simulink library "Quat2Euler"  (Simulink 7.2)
settings: Solver=ode45  StartTime=0.0  StopTime=10.0  RelTol=1e-3
settings Model: Creator=matlab  LastModifiedBy=matlab

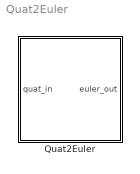
== system Quat2Euler ==
  Quat2Euler : Subsystem  mask(Quat2Euler){euler_order=321, quat_convention=1}
      mask prompts: euler_order "Euler angle order"; quat_convention "Quaternion scalar convention"
      mask help: Convert quaternion to Euler angles
      mask StyleString: popup(312|321|123|132|231|213|121|131|212|232|313|323),popup(1|4)

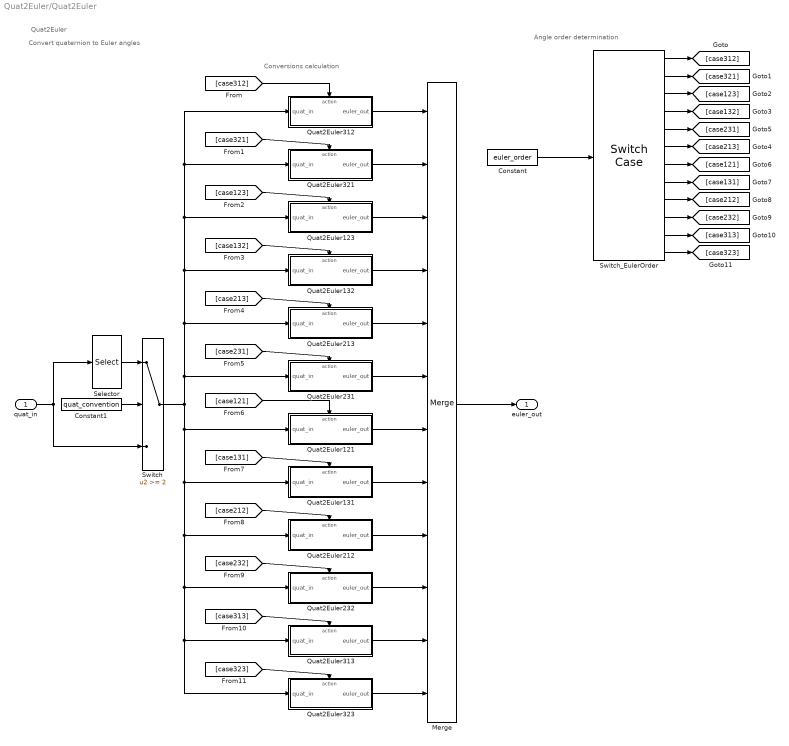
== system Quat2Euler/Quat2Euler ==
  note: Quat2Euler
  note: Convert quaternion to Euler angles
  note: Angle order determination
  note: Conversions calculation
  quat_in : Inport  Description=[ ]: Input quaternion.  PortDimensions=4  OutDataType=sfix(16)  OutScaling=2^0
  Constant : Constant  Value=euler_order  OutDataType=sfix(16)  OutScaling=2^0
  Constant1 : Constant  Value=quat_convention  OutDataType=sfix(16)  OutScaling=2^0
  Merge : Merge  Inputs=12
  Quat2Euler121 : Subsystem  TreatAsAtomicUnit=on
  Quat2Euler123 : Subsystem  TreatAsAtomicUnit=on
  Quat2Euler131 : Subsystem  TreatAsAtomicUnit=on
  Quat2Euler132 : Subsystem  TreatAsAtomicUnit=on
  Quat2Euler212 : Subsystem  TreatAsAtomicUnit=on
  Quat2Euler213 : Subsystem  TreatAsAtomicUnit=on
  Quat2Euler231 : Subsystem  TreatAsAtomicUnit=on
  Quat2Euler232 : Subsystem  TreatAsAtomicUnit=on
  Quat2Euler312 : Subsystem  TreatAsAtomicUnit=on
  Quat2Euler313 : Subsystem  TreatAsAtomicUnit=on
  Quat2Euler321 : Subsystem  TreatAsAtomicUnit=on
  Quat2Euler323 : Subsystem  TreatAsAtomicUnit=on
  Selector : Selector  InputPortWidth=4  IndexOptions=Index vector (dialog)  Indices=[4 1 2 3]  OutputSizes=1
  Switch : Switch  Threshold=2  OutDataType=sfix(16)  OutScaling=2^0
  Switch_EulerOrder : SwitchCase  CaseConditions={1,2,3,4,5,6,7,8,9,10,11,12}  CaseShowDefault=off
  euler_out : Outport  Description=[rad]: Eqivalent Euler angles.  PortDimensions=3  OutDataType=sfix(16)  OutScaling=2^0
  wires:
  Merge/1 -> euler_out/1
  Switch/1 -> Quat2Euler121/1(quat_in), Quat2Euler131/1(quat_in), Quat2Euler212/1(quat_in), Quat2Euler232/1(quat_in), Quat2Euler323/1(quat_in), Quat2Euler313/1(quat_in), Quat2Euler231/1(quat_in), Quat2Euler213/1(quat_in), Quat2Euler132/1(quat_in), Quat2Euler123/1(quat_in), Quat2Euler321/1(quat_in), Quat2Euler312/1(quat_in)
  quat_in/1 -> Switch/3, Selector/1
  Constant1/1 -> Switch/2
  Selector/1 -> Switch/1
  Quat2Euler121/1(euler_out) -> Merge/7
  Quat2Euler312/1(euler_out) -> Merge/1
  Quat2Euler321/1(euler_out) -> Merge/2
  Quat2Euler123/1(euler_out) -> Merge/3
  Quat2Euler132/1(euler_out) -> Merge/4
  Quat2Euler213/1(euler_out) -> Merge/5
  Quat2Euler231/1(euler_out) -> Merge/6
  Quat2Euler131/1(euler_out) -> Merge/8
  Quat2Euler212/1(euler_out) -> Merge/9
  Quat2Euler232/1(euler_out) -> Merge/10
  Quat2Euler313/1(euler_out) -> Merge/11
  Quat2Euler323/1(euler_out) -> Merge/12
  [case121] -> Quat2Euler121/Action
  [case131] -> Quat2Euler131/Action
  [case212] -> Quat2Euler212/Action
  [case232] -> Quat2Euler232/Action
  [case313] -> Quat2Euler313/Action
  [case323] -> Quat2Euler323/Action
  Switch_EulerOrder/12 -> [case323]
  Switch_EulerOrder/11 -> [case313]
  Switch_EulerOrder/10 -> [case232]
  Switch_EulerOrder/9 -> [case212]
  Switch_EulerOrder/8 -> [case131]
  Switch_EulerOrder/7 -> [case121]
  Switch_EulerOrder/5 -> [case231]
  Switch_EulerOrder/6 -> [case213]
  Constant/1 -> Switch_EulerOrder/1
  Switch_EulerOrder/1 -> [case312]
  Switch_EulerOrder/3 -> [case123]
  Switch_EulerOrder/2 -> [case321]
  Switch_EulerOrder/4 -> [case132]
  [case312] -> Quat2Euler312/Action
  [case321] -> Quat2Euler321/Action
  [case123] -> Quat2Euler123/Action
  [case132] -> Quat2Euler132/Action
  [case213] -> Quat2Euler213/Action
  [case231] -> Quat2Euler231/Action

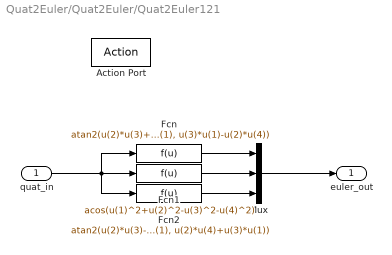
== system Quat2Euler/Quat2Euler/Quat2Euler121 ==
  quat_in : Inport  OutDataType=sfix(16)  OutScaling=2^0
  Action Port : ActionPort
  Fcn : Fcn  Expr=atan2(u(2)*u(3)+u(4)*u(1), u(3)*u(1)-u(2)*u(4))
  Fcn1 : Fcn  Expr=acos(u(1)^2+u(2)^2-u(3)^2-u(4)^2)
  Fcn2 : Fcn  Expr=atan2(u(2)*u(3)-u(4)*u(1), u(2)*u(4)+u(3)*u(1))
  Mux : Mux  Inputs=3
  euler_out : Outport  OutDataType=sfix(16)  OutScaling=2^0
  wires:
  Mux/1 -> euler_out/1
  quat_in/1 -> Fcn2/1, Fcn/1, Fcn1/1
  Fcn2/1 -> Mux/3
  Fcn1/1 -> Mux/2
  Fcn/1 -> Mux/1

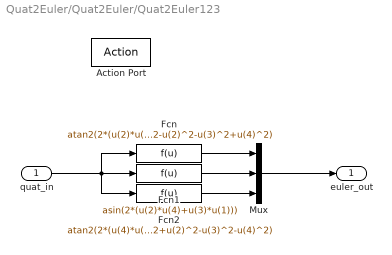
== system Quat2Euler/Quat2Euler/Quat2Euler123 ==
  quat_in : Inport  OutDataType=sfix(16)  OutScaling=2^0
  Action Port : ActionPort
  Fcn : Fcn  Expr=atan2(2*(u(2)*u(1)-u(3)*u(4)),u(1)^2-u(2)^2-u(3)^2+u(4)^2)
  Fcn1 : Fcn  Expr=asin(2*(u(2)*u(4)+u(3)*u(1)))
  Fcn2 : Fcn  Expr=atan2(2*(u(4)*u(1)-u(2)*u(3)),u(1)^2+u(2)^2-u(3)^2-u(4)^2)
  Mux : Mux  Inputs=3
  euler_out : Outport  OutDataType=sfix(16)  OutScaling=2^0
  wires:
  Mux/1 -> euler_out/1
  quat_in/1 -> Fcn2/1, Fcn/1, Fcn1/1
  Fcn2/1 -> Mux/3
  Fcn1/1 -> Mux/2
  Fcn/1 -> Mux/1

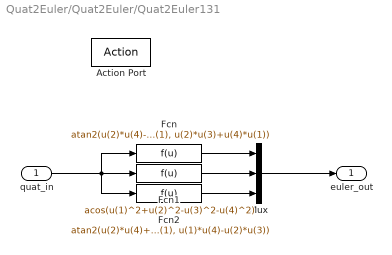
== system Quat2Euler/Quat2Euler/Quat2Euler131 ==
  quat_in : Inport  OutDataType=sfix(16)  OutScaling=2^0
  Action Port : ActionPort
  Fcn : Fcn  Expr=atan2(u(2)*u(4)-u(3)*u(1), u(2)*u(3)+u(4)*u(1))
  Fcn1 : Fcn  Expr=acos(u(1)^2+u(2)^2-u(3)^2-u(4)^2)
  Fcn2 : Fcn  Expr=atan2(u(2)*u(4)+u(3)*u(1), u(1)*u(4)-u(2)*u(3))
  Mux : Mux  Inputs=3
  euler_out : Outport  OutDataType=sfix(16)  OutScaling=2^0
  wires:
  Fcn/1 -> Mux/1
  Fcn1/1 -> Mux/2
  Fcn2/1 -> Mux/3
  quat_in/1 -> Fcn1/1, Fcn/1, Fcn2/1
  Mux/1 -> euler_out/1

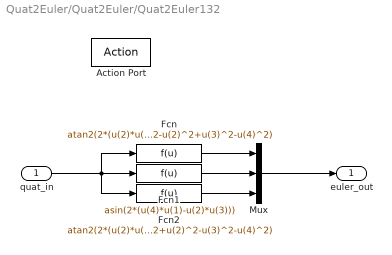
== system Quat2Euler/Quat2Euler/Quat2Euler132 ==
  quat_in : Inport  OutDataType=sfix(16)  OutScaling=2^0
  Action Port : ActionPort
  Fcn : Fcn  Expr=atan2(2*(u(2)*u(1)+u(3)*u(4)),u(1)^2-u(2)^2+u(3)^2-u(4)^2)
  Fcn1 : Fcn  Expr=asin(2*(u(4)*u(1)-u(2)*u(3)))
  Fcn2 : Fcn  Expr=atan2(2*(u(2)*u(4)+u(3)*u(1)),u(1)^2+u(2)^2-u(3)^2-u(4)^2)
  Mux : Mux  Inputs=3
  euler_out : Outport  OutDataType=sfix(16)  OutScaling=2^0
  wires:
  Fcn/1 -> Mux/1
  Fcn1/1 -> Mux/2
  Fcn2/1 -> Mux/3
  quat_in/1 -> Fcn1/1, Fcn/1, Fcn2/1
  Mux/1 -> euler_out/1

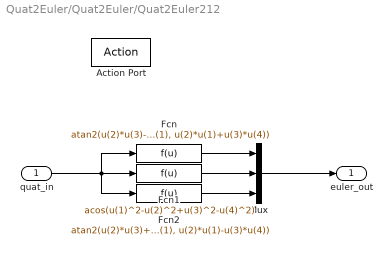
== system Quat2Euler/Quat2Euler/Quat2Euler212 ==
  quat_in : Inport  OutDataType=sfix(16)  OutScaling=2^0
  Action Port : ActionPort
  Fcn : Fcn  Expr=atan2(u(2)*u(3)-u(4)*u(1), u(2)*u(1)+u(3)*u(4))
  Fcn1 : Fcn  Expr=acos(u(1)^2-u(2)^2+u(3)^2-u(4)^2)
  Fcn2 : Fcn  Expr=atan2(u(2)*u(3)+u(4)*u(1), u(2)*u(1)-u(3)*u(4))
  Mux : Mux  Inputs=3
  euler_out : Outport  OutDataType=sfix(16)  OutScaling=2^0
  wires:
  Mux/1 -> euler_out/1
  quat_in/1 -> Fcn2/1, Fcn/1, Fcn1/1
  Fcn2/1 -> Mux/3
  Fcn1/1 -> Mux/2
  Fcn/1 -> Mux/1

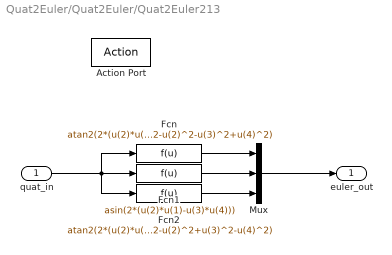
== system Quat2Euler/Quat2Euler/Quat2Euler213 ==
  quat_in : Inport  OutDataType=sfix(16)  OutScaling=2^0
  Action Port : ActionPort
  Fcn : Fcn  Expr=atan2(2*(u(2)*u(4)+u(3)*u(1)),u(1)^2-u(2)^2-u(3)^2+u(4)^2)
  Fcn1 : Fcn  Expr=asin(2*(u(2)*u(1)-u(3)*u(4)))
  Fcn2 : Fcn  Expr=atan2(2*(u(2)*u(3)+u(4)*u(1)),u(1)^2-u(2)^2+u(3)^2-u(4)^2)
  Mux : Mux  Inputs=3
  euler_out : Outport  OutDataType=sfix(16)  OutScaling=2^0
  wires:
  Mux/1 -> euler_out/1
  quat_in/1 -> Fcn2/1, Fcn/1, Fcn1/1
  Fcn2/1 -> Mux/3
  Fcn1/1 -> Mux/2
  Fcn/1 -> Mux/1

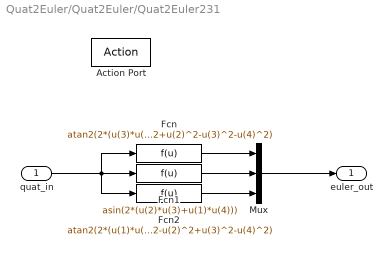
== system Quat2Euler/Quat2Euler/Quat2Euler231 ==
  quat_in : Inport  OutDataType=sfix(16)  OutScaling=2^0
  Action Port : ActionPort
  Fcn : Fcn  Expr=atan2(2*(u(3)*u(1)-u(4)*u(2)),u(1)^2+u(2)^2-u(3)^2-u(4)^2)
  Fcn1 : Fcn  Expr=asin(2*(u(2)*u(3)+u(1)*u(4)))
  Fcn2 : Fcn  Expr=atan2(2*(u(1)*u(2)-u(3)*u(4)),u(1)^2-u(2)^2+u(3)^2-u(4)^2)
  Mux : Mux  Inputs=3
  euler_out : Outport  OutDataType=sfix(16)  OutScaling=2^0
  wires:
  Fcn/1 -> Mux/1
  Fcn1/1 -> Mux/2
  Fcn2/1 -> Mux/3
  quat_in/1 -> Fcn1/1, Fcn/1, Fcn2/1
  Mux/1 -> euler_out/1

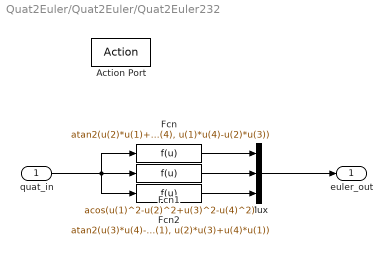
== system Quat2Euler/Quat2Euler/Quat2Euler232 ==
  quat_in : Inport  OutDataType=sfix(16)  OutScaling=2^0
  Action Port : ActionPort
  Fcn : Fcn  Expr=atan2(u(2)*u(1)+u(3)*u(4), u(1)*u(4)-u(2)*u(3))
  Fcn1 : Fcn  Expr=acos(u(1)^2-u(2)^2+u(3)^2-u(4)^2)
  Fcn2 : Fcn  Expr=atan2(u(3)*u(4)-u(2)*u(1), u(2)*u(3)+u(4)*u(1))
  Mux : Mux  Inputs=3
  euler_out : Outport  OutDataType=sfix(16)  OutScaling=2^0
  wires:
  Fcn/1 -> Mux/1
  Fcn1/1 -> Mux/2
  Fcn2/1 -> Mux/3
  quat_in/1 -> Fcn1/1, Fcn/1, Fcn2/1
  Mux/1 -> euler_out/1

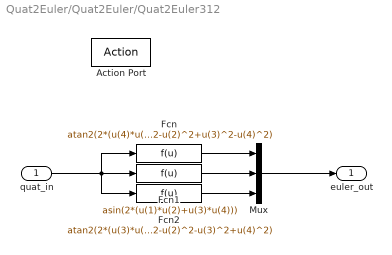
== system Quat2Euler/Quat2Euler/Quat2Euler312 ==
  quat_in : Inport  OutDataType=sfix(16)  OutScaling=2^0
  Action Port : ActionPort
  Fcn : Fcn  Expr=atan2(2*(u(4)*u(1)-u(2)*u(3)),u(1)^2-u(2)^2+u(3)^2-u(4)^2)
  Fcn1 : Fcn  Expr=asin(2*(u(1)*u(2)+u(3)*u(4)))
  Fcn2 : Fcn  Expr=atan2(2*(u(3)*u(1)-u(2)*u(4)),u(1)^2-u(2)^2-u(3)^2+u(4)^2)
  Mux : Mux  Inputs=3
  euler_out : Outport  OutDataType=sfix(16)  OutScaling=2^0
  wires:
  Mux/1 -> euler_out/1
  quat_in/1 -> Fcn2/1, Fcn/1, Fcn1/1
  Fcn2/1 -> Mux/3
  Fcn1/1 -> Mux/2
  Fcn/1 -> Mux/1

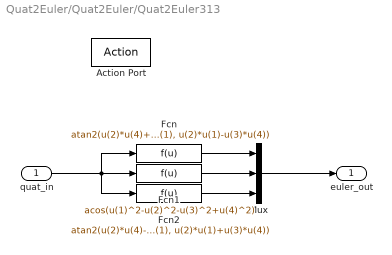
== system Quat2Euler/Quat2Euler/Quat2Euler313 ==
  quat_in : Inport  OutDataType=sfix(16)  OutScaling=2^0
  Action Port : ActionPort
  Fcn : Fcn  Expr=atan2(u(2)*u(4)+u(3)*u(1), u(2)*u(1)-u(3)*u(4))
  Fcn1 : Fcn  Expr=acos(u(1)^2-u(2)^2-u(3)^2+u(4)^2)
  Fcn2 : Fcn  Expr=atan2(u(2)*u(4)-u(3)*u(1), u(2)*u(1)+u(3)*u(4))
  Mux : Mux  Inputs=3
  euler_out : Outport  OutDataType=sfix(16)  OutScaling=2^0
  wires:
  Mux/1 -> euler_out/1
  quat_in/1 -> Fcn2/1, Fcn/1, Fcn1/1
  Fcn2/1 -> Mux/3
  Fcn1/1 -> Mux/2
  Fcn/1 -> Mux/1

== system Quat2Euler/Quat2Euler/Quat2Euler321 ==
  quat_in : Inport  OutDataType=sfix(16)  OutScaling=2^0
  Action Port : ActionPort
  Fcn : Fcn  Expr=atan2(2*(u(2)*u(3)+u(4)*u(1)),u(1)^2+u(2)^2-u(3)^2-u(4)^2)
  Fcn1 : Fcn  Expr=asin(2*(u(3)*u(1)-u(2)*u(4)))
  Fcn2 : Fcn  Expr=atan2(2*(u(2)*u(1)+u(4)*u(3)),u(1)^2-u(2)^2-u(3)^2+u(4)^2)
  Mux : Mux  Inputs=3
  euler_out : Outport  OutDataType=sfix(16)  OutScaling=2^0
  wires:
  Fcn/1 -> Mux/1
  Fcn1/1 -> Mux/2
  Fcn2/1 -> Mux/3
  quat_in/1 -> Fcn1/1, Fcn/1, Fcn2/1
  Mux/1 -> euler_out/1

== system Quat2Euler/Quat2Euler/Quat2Euler323 ==
  quat_in : Inport  OutDataType=sfix(16)  OutScaling=2^0
  Action Port : ActionPort
  Fcn : Fcn  Expr=atan2(u(3)*u(4)-u(1)*u(2), u(2)*u(4)+u(3)*u(1))
  Fcn1 : Fcn  Expr=acos(u(1)^2-u(2)^2-u(3)^2+u(4)^2)
  Fcn2 : Fcn  Expr=atan2(u(2)*u(1)+u(3)*u(4), u(3)*u(1)-u(2)*u(4))
  Mux : Mux  Inputs=3
  euler_out : Outport  OutDataType=sfix(16)  OutScaling=2^0
  wires:
  Fcn/1 -> Mux/1
  Fcn1/1 -> Mux/2
  Fcn2/1 -> Mux/3
  quat_in/1 -> Fcn1/1, Fcn/1, Fcn2/1
  Mux/1 -> euler_out/1
